simulink model "SKKPmdl"  (Simulink 8.4)
settings: Solver=ode113  StartTime=0.0  StopTime=900  FixedStep=0.1  RelTol=1e-1  AbsTol=1e-1
undefined symbols (not defined in the file or in its folder): deg, eps_max, eps_min, H3dm, H4dm, Jdm, L, M3dm, M4dm, Newton, P, R0, rad, Raphson, s, Td, Tpp, V0, y_out
libraries: aerolibconvert2 x26, aerolibtransform2 x19, aerolibutil x7, aerolibobsolete x6, dspinverses x5, vrlib x1, aerolib6dof2 x1
(part 1 of 2)
settings Model: Creator=Mikhail  LastModifiedBy=Mikhail  PauseTimes=1  BufferReuse=off
settings DataIOCC: SignalLoggingSaveFormat=Dataset
settings OptimizationCC: BlockReduction=off  InlineParams=on  BufferReuse=off  ExpressionDepthLimit=128
settings DebuggingCC: UnderspecifiedInitializationDetection=Simplified  MergeDetectMultiDrivingBlocksExec=error  FcnCallInpInsideContextMsg=EnableAllAsError  StateNameClashWarn=none
settings GRTTargetCC: CombineOutputUpdateFcns=on  GRTInterface=off

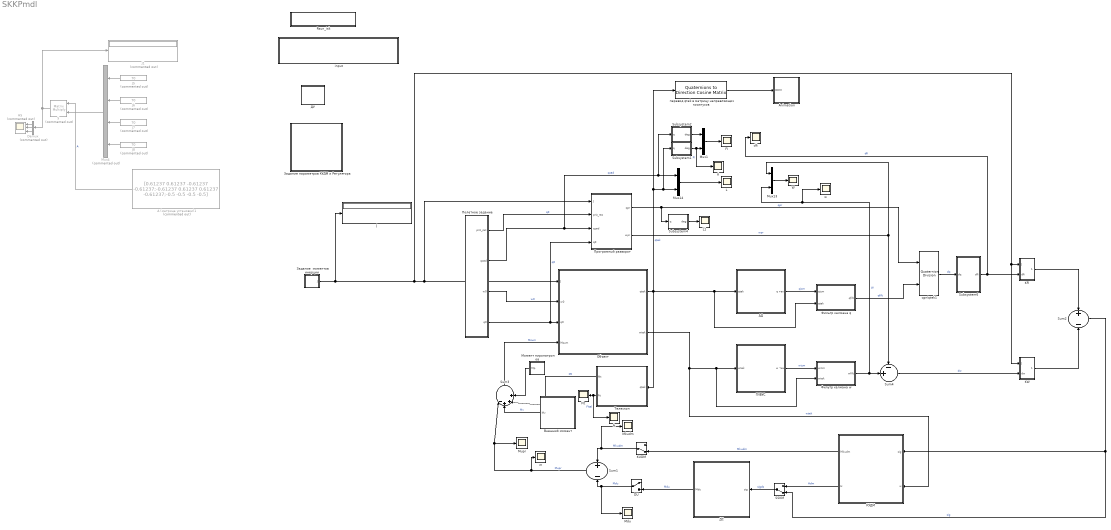
== system SKKPmdl ==
  " 5" : Product  Commented=on  Multiplication=Matrix(*)
  Animation : Subsystem  AncestorBlock=aerolibanim/6DoF Animation  mask(Animation){u2=10, u8=off}
      mask prompts: u2 "Time interval between updates:"; u8 "Enable animation"
      mask help: Create a 3-D animated.
      mask init:
      | Config.update = u2;
      | Config.Animenable = u8;
      mask Help: web(asbhelp('6dofanimation'));
  DU : ManualSwitch
  Demux : Demux  Commented=on  Outputs=3
  FI : Scope
      settings: TickLabels=on  YMax=30  SaveName=FI  SampleInput=on  ScrollMode=on
  FIt : Scope
      settings: YMin=-20  YMax=100  SaveName=FIt
  H5 : Scope  Commented=on  NumInputPorts=3
      settings: TimeRange=250  YMin=-100~-5~-5  YMax=600~5~5  SaveName=H4dm3
  J : Display
  J1 : Display  Commented=on
  J{5..8} (4 alike) : Constant  Commented=on  Value=70
  KFI : Subsystem
  KUDM : ManualSwitch  CurrentSetting=0
  KW : Subsystem
  L : Scope
      settings: YMin=0  YMax=1  SaveName=L
  L1 : Scope
      settings: YMin=0  YMax=8  SaveName=L1
  Mdu : Scope
      settings: YMin=-0.2  YMax=1  SaveName=Mdu
  Mkudm : Scope
      settings: YMin=-0.25  YMax=0.05  SaveName=Mkudm
  Mupr : Scope
      settings: YMin=-0.1  YMax=0.6  SaveName=Mupr
  Mux1 : Mux  Inputs=2
  Mux13 : Mux  Inputs=2
  Mux14 : Mux  Inputs=2
  Mux4 : Mux  Commented=on
  "Rsun_isk " : Subsystem  mask{rsun=[3 50 0]'}
      mask init:
      | Rsun=rsun/(norm(rsun));
      | assignin('base','Rsun',Rsun);
      | st=sprintf('Rsun=[%1.2g %1.2g %1.2g]\n',Rsun);
      mask Display: disp(st);
  SSKM : ManualSwitch  CurrentSetting=0
  Subsystem1 : Subsystem
  Subsystem2 : Subsystem
  Subsystem4 : Subsystem
  Subsystem6 : Subsystem
  Sum1 : Sum  Inputs=+-
  Sum2 : Sum  Inputs=+-
  Sum3 : Sum  Inputs=|-+++
  Sum4 : Sum  Inputs=-+|
  W : Scope
      settings: TimeRange=350  YMin=-50  YMax=250  SaveName=W
  dfi : Scope
      settings: YMin=-0.2  YMax=0.1  SaveName=dfi
  fi : Scope
      settings: ShowLegends=on  YMax=35  SaveName=ScopeData2
  ft : Scope
      settings: ShowLegends=on  YMin=-50  YMax=200  SaveName=ScopeData8
  input : Subsystem  mask{P=1, L=1.5, Td=0.1, X=0.006, Y=1.229, Z=-0.001}
      mask init:
      | assignin('base','P',P);
      | assignin('base','L',L);
      | assignin('base','Td',Td);
      | assignin('base','X',X);
      | assignin('base','Y',Y);
      | assignin('base','Z',Z);
      | 
      | st=sprintf('Тяга P =%1.3fН\n Плечо L =%1.3fм\n Постоянная времени нарастания/спада  Td =%1.3fc\n',P,L,Td);
      mask Callback P:
      | %assignin('base','psi0',psi0);
      | %assignin('base','tetta0',tetta0);
      mask Display: disp(st);
  m : Scope
      settings: ShowLegends=on  TimeRange=14.16568047337279  YMin=0.2  YMax=0.45  SaveName=ScopeData7
  qpr/qtek1 : aerolibutil/Quaternion Division
  w : Scope
      settings: ShowLegends=on  YMin=0  YMax=0.2  SaveName=ScopeData5
  А (матрица установки)1 : Constant  Commented=on  Value=[0.61237 0.61237 -0.61237 -0.61237;-0.61237 0.61237 0.61237 -0.61237;-0.5 -0.5 -0.5 -0.5]
  АД : Subsystem
      mask Display: image(imread('AD.png'))
  Внешний момент : Subsystem
  ГИВУС : Subsystem
      mask Display: image(imread('GIVUS.jpg'))
  ДC : Subsystem
      mask Display: image(imread('DS.jpg'))
  ДУ : Subsystem  mask{eps_min=1, eps_max=0.1, y_out=1}
      mask prompts: eps_min "Порог включения"; eps_max "Порог отключения"; y_out "Выходной сигнал"
      mask init:
      | assignin('base','eps_min',eps_min);
      | assignin('base','eps_max',eps_max);
      | assignin('base','y_out',y_out);
      mask Display:
      | plot([0.1 0.9],[0.5 0.5]);
      | plot([0.5 0.5],[0.1 0.9]);
      | plot([0.1 0.4 0.4 0.6 0.6 0.9],[0.3 0.3 0.5 0.5 0.7 0.7])
      | plot([0.1 0.45 0.45 0.55 0.55 0.9],[0.3 0.3 0.5 0.5 0.7 0.7])
  Задание  моментов инерции : Subsystem
  Задание параметров КУДМ и Регулятора : Subsystem  mask{jdm=0.0634646, tpp=50, e=0.8, m3dm=0.3, m4dm=0.4, h3dm=43, h4dm=140}
      mask init:
      | Jdm=jdm;
      | Tpp=tpp;
      | E=e;
      | M3dm=m3dm;
      | M4dm=m4dm;
      | H3dm=h3dm;
      | H4dm=h4dm;
      | 
      | assignin('base','Jdm',Jdm);
      | 
      | assignin('base','Tpp',Tpp);
      | assignin('base','E',E);
      | 
      | assignin('base','M3dm',M3dm);
      | assignin('base','M4dm',M4dm);
      | 
      | assignin('base','H3dm',H3dm);
      | assignin('base','H4dm',H4dm);
      | 
      | st=sprintf('Jdm=%g\n Tpp=%g\n E=%g\n M3dm=%g\n M4dm=%g\n H3dm=%g\n H4dm=%g\n',jdm,tpp,e,m3dm,m4dm,h3dm,h4dm);
      mask Display: disp(st);
  КУДМ : Subsystem
      mask Display: image(imread('KUDM.jpg'))
  Момент пиропатронов : Subsystem
  Объект : Subsystem
      mask Display: image(imread('КА.png'))
  Полетное задание : Subsystem
  "Програмный разворот " : Subsystem
  Телескоп : Subsystem
      mask Display: image(imread('Tel.png'))
  "Фильтр калмана q " : Subsystem
  "Фильтр калмана w " : Subsystem
  "перевод qtek в матрицу направляющих косинусов " : aerolibtransform2/Quaternions to  Direction Cosine Matrix
  wires:
  "Програмный разворот "/1(qpr) -> Subsystem4/1(q), qpr/qtek1/1  "qpr"
  Объект/2(wtek) -> КУДМ/2(w), "Фильтр калмана w "/2(wtek), ГИВУС/1(wtek)  "wtek"
  ГИВУС/1(w тек) -> "Фильтр калмана w "/1(wizm)  "wizm"
  Объект/1(qtek) -> "Фильтр калмана q "/2(qtek), АД/1("qtek "), Телескоп/1(qtek), "перевод qtek в матрицу направляющих косинусов "/1, Subsystem1/1(q), Mux14/2  "qtek"
  АД/1(q тек) -> "Фильтр калмана q "/1(qizm)  "qizm"
  Полетное задание/3(w0) -> Объект/2(w0)  "w0"
  qpr/qtek1/1 -> Subsystem6/1(dq)  "dq"
  Subsystem6/1(dfi) -> dfi/1, KFI/2(dfi)  "dfi"
  Sum2/1 -> SSKM/2, КУДМ/1(sig)  "sig"
  КУДМ/2(H) -> SSKM/1  "Hdm"
  SSKM/1 -> ДC/1(sig)  "sigds"
  ДC/1(Mdu) -> DU/2  "Mdu"
  КУДМ/1(Mkudm) -> KUDM/2  "Mkudm"
  Внешний момент/1("Mv ") -> Sum3/2  "Mv"
  Sum1/1 -> m/1, Mupr/1, Sum3/1  "Mupr"
  Sum3/1 -> Объект/4(Msum)  "Msum"
  "Фильтр калмана q "/1(qfilt) -> qpr/qtek1/2  "qfilt"
  Mux14/1 -> L/1
  "Програмный разворот "/2(wpr) -> Sum4/1, Mux13/1  "wpr"
  Mux13/1 -> W/1
  "Фильтр калмана w "/1(wfilt) -> w/1, Mux13/2, Sum4/2  "W"
  KUDM/1 -> Mkudm/1, Sum1/1  "Mkudm"
  DU/1 -> Mdu/1, Sum1/2  "Mdu"
  Subsystem1/1(deg) -> fi/1, Mux1/2  "FI"
  Subsystem2/1(deg) -> Mux1/1
  Mux1/1 -> FI/1
  "перевод qtek в матрицу направляющих косинусов "/1 -> Animation/1(DCM)
  Полетное задание/4(q0) -> "Програмный разворот "/4(q0), Объект/3("q0 ")  "q0"
  Subsystem4/1(deg) -> L1/1
  Полетное задание/1(priz_raz) -> "Програмный разворот "/2(priz_raz)  "q0"
  Полетное задание/2(qzad) -> Subsystem2/1(q), Mux14/1, "Програмный разворот "/3(qzad)  "qzad"
  Телескоп/1(Mt) -> Sum3/3  "Mt"
  Телескоп/2(fit) -> ft/1, FIt/1  "FItel"
  Задание  моментов инерции/1(J) -> "Програмный разворот "/1(J), Объект/1(J), KW/1(J), KFI/1(J), J/1
  Момент пиропатронов/1(Mp) -> Sum3/4
  KFI/1(kfi*dfi) -> Sum2/1
  Sum4/1 -> KW/2(dw)  "dw"
  KW/1(kw*dw) -> Sum2/2
  J5/1 -> Mux4/1
  J6/1 -> Mux4/2
  J7/1 -> Mux4/3
  J8/1 -> Mux4/4
  Mux4/1 -> " 5"/2
  " 5"/1 -> Demux/1, J1/1
  Demux/1 -> H5/1
  Demux/2 -> H5/2
  Demux/3 -> H5/3
  А (матрица установки)1/1 -> " 5"/1  "A"

== system SKKPmdl/Animation ==
  DCM : Inport
  Animation S-Function : S-Function  FunctionName=saeroanim  Parameters=Config  EnableBusSupport=off
  Reshape : Reshape
  wires:
  DCM/1 -> Reshape/1
  Reshape/1 -> Animation S-Function/1

== system SKKPmdl/KFI ==
  J : Inport
  dfi : Inport  Port=2
  Demux : Demux  Outputs=9
  Display4 : Display
  Divide1 : Product  Inputs=**
  Divide3 : Product  Inputs=/*
  Divide4 : Product  Inputs=/*
  Divide5 : Product  Inputs=/*
  Mux : Mux  Inputs=3
  Reshape : Reshape  OutputDimensionality=Column vector (2-D)
  eps_max3 : Constant  Value=Tpp*Tpp
  kfi*dfi : Outport
  wires:
  Divide1/1 -> kfi*dfi/1  "kfi*dfi"
  Demux/5 -> Divide4/2
  eps_max3/1 -> Divide5/1, Divide4/1, Divide3/1
  Demux/9 -> Divide5/2
  Divide3/1 -> Mux/1
  Divide4/1 -> Mux/2
  Divide5/1 -> Mux/3
  Demux/1 -> Divide3/2
  Reshape/1 -> Demux/1
  Mux/1 -> Divide1/1, Display4/1
  dfi/1 -> Divide1/2
  J/1 -> Reshape/1

== system SKKPmdl/KW ==
  J : Inport
  dw : Inport  Port=2
  Demux1 : Demux  Outputs=9
  Display5 : Display
  Divide{2,6..8} (4 alike) : Product  Inputs=**
  Mux2 : Mux  Inputs=3
  Reshape1 : Reshape  OutputDimensionality=Column vector (2-D)
  eps_max1 : Constant  Value=(2*E)/Tpp
  kw*dw : Outport
  wires:
  dw/1 -> Divide2/2
  Divide2/1 -> kw*dw/1  "kw*dw"
  Demux1/1 -> Divide6/2
  Demux1/9 -> Divide8/2
  eps_max1/1 -> Divide6/1, Divide7/1, Divide8/1
  Demux1/5 -> Divide7/2
  Divide6/1 -> Mux2/1
  Divide7/1 -> Mux2/2
  Divide8/1 -> Mux2/3
  Reshape1/1 -> Demux1/1
  Mux2/1 -> Display5/1, Divide2/1
  J/1 -> Reshape1/1

== system SKKPmdl/Rsun_isk  ==

== system SKKPmdl/Subsystem1 ==
  q : Inport
  Angle Conversion1 : aerolibconvert2/Angle Conversion  IU=rad  OU=deg
  Direction Cosine Matrix to Euler Angles1 : aerolibobsolete/Direction Cosine Matrix to Euler Angles
  Quaternions to  Direction Cosine Matrix3 : aerolibtransform2/Quaternions to  Direction Cosine Matrix
  deg : Outport
  wires:
  Quaternions to  Direction Cosine Matrix3/1 -> Direction Cosine Matrix to Euler Angles1/1
  Direction Cosine Matrix to Euler Angles1/1 -> Angle Conversion1/1
  Angle Conversion1/1 -> deg/1
  q/1 -> Quaternions to  Direction Cosine Matrix3/1

== system SKKPmdl/Subsystem2 ==
  q : Inport
  Angle Conversion1 : aerolibconvert2/Angle Conversion  IU=rad  OU=deg
  Direction Cosine Matrix to Euler Angles1 : aerolibobsolete/Direction Cosine Matrix to Euler Angles
  Quaternions to  Direction Cosine Matrix3 : aerolibtransform2/Quaternions to  Direction Cosine Matrix
  deg : Outport
  wires:
  q/1 -> Quaternions to  Direction Cosine Matrix3/1
  Angle Conversion1/1 -> deg/1
  Direction Cosine Matrix to Euler Angles1/1 -> Angle Conversion1/1
  Quaternions to  Direction Cosine Matrix3/1 -> Direction Cosine Matrix to Euler Angles1/1

== system SKKPmdl/Subsystem4 ==
  q : Inport
  Angle Conversion1 : aerolibconvert2/Angle Conversion  IU=rad  OU=deg
  Direction Cosine Matrix to Euler Angles1 : aerolibobsolete/Direction Cosine Matrix to Euler Angles
  Quaternions to  Direction Cosine Matrix3 : aerolibtransform2/Quaternions to  Direction Cosine Matrix
  deg : Outport
  wires:
  Quaternions to  Direction Cosine Matrix3/1 -> Direction Cosine Matrix to Euler Angles1/1
  Direction Cosine Matrix to Euler Angles1/1 -> Angle Conversion1/1
  Angle Conversion1/1 -> deg/1
  q/1 -> Quaternions to  Direction Cosine Matrix3/1

== system SKKPmdl/Subsystem6 ==
  dq : Inport
  Angle C5 : aerolibconvert2/Angle Conversion  IU=rad  OU=deg
  Перевод из матрицы направляющих косинусов  в dfi1 : aerolibobsolete/Direction Cosine Matrix to Euler Angles
  перевод dq в матрицу направляющих косинусов 1 : aerolibtransform2/Quaternions to  Direction Cosine Matrix
  dfi : Outport
  wires:
  перевод dq в матрицу направляющих косинусов 1/1 -> Перевод из матрицы направляющих косинусов  в dfi1/1  "DCM"
  dq/1 -> перевод dq в матрицу направляющих косинусов 1/1
  Перевод из матрицы направляющих косинусов  в dfi1/1 -> Angle C5/1  "dfi"
  Angle C5/1 -> dfi/1

== system SKKPmdl/input ==

== system SKKPmdl/АД ==
  "qtek " : Inport
  Gain3 : Gain  Gain=3
  Gain4 : Gain  Gain=3
  Gain5 : Gain  Gain=3
  Mux2 : Mux  Inputs=3
  Noise1____5''1 : RandomNumber  Variance=0.0013888888888889  Seed=23456
  Noise2___5''1 : RandomNumber  Variance=0.0013888888888889  Seed=23455
  Noise3___5''1 : RandomNumber  Variance=0.0013888888888889  Seed=23457
  Quaternion Multiplication3 : aerolibutil/Quaternion Multiplication
  Quaternion Multiplication4 : aerolibutil/Quaternion Multiplication
  Quaternion Multiplication5 : aerolibutil/Quaternion Multiplication
  Zero-Order Hold8 : ZeroOrderHold  SampleTime=0.1
  Мвск-пск 1 : Constant  Value=[0 0 1;-0.5 0.87 0;-0.87 -0.5 0]
  Мпск-вск1 : Constant  Value=[0 -0.5 -0.85; 0 0.85 -0.5; 1 0 0]
  Перевод из матрицы  направляющих  косинусов в  кватернионы2 : aerolibtransform2/Direction Cosine Matrix  to Quaternions
  Перевод из матрицы  направляющих  косинусов в  кватернионы3 : aerolibtransform2/Direction Cosine Matrix  to Quaternions
  Перевод из углов  в кватернионы1 : Subsystem
  q тек : Outport
  wires:
  Мвск-пск 1/1 -> Перевод из матрицы  направляющих  косинусов в  кватернионы2/1  "Mвск-пск"
  Noise1____5''1/1 -> Gain3/1
  Noise2___5''1/1 -> Gain4/1
  Noise3___5''1/1 -> Gain5/1
  Mux2/1 -> Перевод из углов  в кватернионы1/1(fi)
  "qtek "/1 -> Quaternion Multiplication3/2  "qtek"
  Перевод из матрицы  направляющих  косинусов в  кватернионы2/1 -> Quaternion Multiplication3/1
  Перевод из углов  в кватернионы1/1(q) -> Quaternion Multiplication4/2  "Добавление шумовой составляющей АД"
  Мпск-вск1/1 -> Перевод из матрицы  направляющих  косинусов в  кватернионы3/1  "Mпск-вск"
  Quaternion Multiplication4/1 -> Quaternion Multiplication5/2
  Quaternion Multiplication5/1 -> q тек/1
  Перевод из матрицы  направляющих  косинусов в  кватернионы3/1 -> Quaternion Multiplication5/1
  Gain3/1 -> Mux2/1
  Gain4/1 -> Mux2/2
  Gain5/1 -> Mux2/3
  Quaternion Multiplication3/1 -> Quaternion Multiplication4/1

== system SKKPmdl/Внешний момент ==
  M_vn4 : Step  Time=0  After=0.00001  SampleTime=0
  M_vn5 : Step  Time=0  After=0.00008  SampleTime=0
  M_vn6 : Step  Time=0  After=0.00006  SampleTime=0
  Mux4 : Mux  Inputs=3
  "Mv " : Outport
  wires:
  M_vn4/1 -> Mux4/1
  M_vn6/1 -> Mux4/3
  M_vn5/1 -> Mux4/2
  Mux4/1 -> "Mv "/1

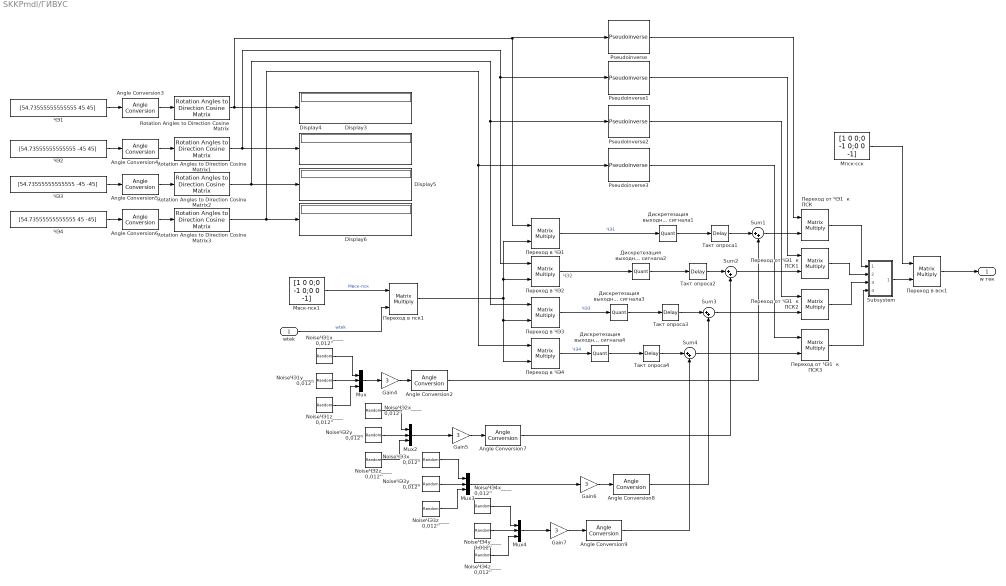
== system SKKPmdl/ГИВУС ==
  note: ЧЭ2
  wtek : Inport
  Angle Conversion{2..9} (8 alike) : aerolibconvert2/Angle Conversion  IU=deg  OU=rad
  Display{3..6} (4 alike) : Display
  Gain{4..7} (4 alike) : Gain  Gain=3
  Mux{,2..4} (4 alike) : Mux  Inputs=3
  NoiseЧЭ1x____0,012'' : RandomNumber  Variance=0.0000033333333333333  Seed=23456
  NoiseЧЭ1y____0,012'' : RandomNumber  Variance=0.0000033333333333333  Seed=23456
  NoiseЧЭ1z____0,012'' : RandomNumber  Variance=0.0000033333333333333  Seed=23456
  NoiseЧЭ2x____0,012'' : RandomNumber  Variance=0.0000033333333333333  Seed=23456
  NoiseЧЭ2y____0,012'' : RandomNumber  Variance=0.0000033333333333333  Seed=23456
  NoiseЧЭ2z____0,012'' : RandomNumber  Variance=0.0000033333333333333  Seed=23456
  NoiseЧЭ3x____0,012'' : RandomNumber  Variance=0.0000033333333333333  Seed=23456
  NoiseЧЭ3y____0,012'' : RandomNumber  Variance=0.0000033333333333333  Seed=23456
  NoiseЧЭ3z____0,012'' : RandomNumber  Variance=0.0000033333333333333  Seed=23456
  NoiseЧЭ4x____0,012'' : RandomNumber  Variance=0.0000033333333333333  Seed=23456
  NoiseЧЭ4y____0,012'' : RandomNumber  Variance=0.0000033333333333333  Seed=23456
  NoiseЧЭ4z____0,012'' : RandomNumber  Variance=0.0000033333333333333  Seed=23456
  Pseudoinverse{,1..3} (4 alike) : dspinverses/Pseudoinverse  wanterr=off
  Rotation Angles to Direction Cosine Matrix{,1..3} (4 alike) : aerolibtransform2/Rotation Angles to Direction Cosine Matrix  rotationOrder=XYZ
  Subsystem : Subsystem
  Sum{1..4} (4 alike) : Sum  Inputs=|++
  Дискретезация выходного сигнала{1..4} (4 alike) : Quantizer  QuantizationInterval=0.000000048481368110954
  Мвск-пск1 : Constant  Value=[1 0 0;0 -1 0;0 0 -1]  VectorParams1D=off
  Мпск-сск : Constant  Value=[1 0 0;0 -1 0;0 0 -1]  VectorParams1D=off
  Переход в ЧЭ{1..4} (4 alike) : Product  Multiplication=Matrix(*)  SaturateOnIntegerOverflow=on  RndMeth=Zero  InputSameDT=on  OutDataTypeStr=Inherit: Same as first input
  Переход в вск1 : Product  Multiplication=Matrix(*)  SaturateOnIntegerOverflow=on  RndMeth=Zero  InputSameDT=on  OutDataTypeStr=Inherit: Same as first input
  Переход в пск1 : Product  Multiplication=Matrix(*)  SaturateOnIntegerOverflow=on  RndMeth=Zero  InputSameDT=on  OutDataTypeStr=Inherit: Same as first input
  Переход от ЧЭ1  к ПСК{,1..3} (4 alike) : Product  Multiplication=Matrix(*)  SaturateOnIntegerOverflow=on  RndMeth=Zero  InputSameDT=on  OutDataTypeStr=Inherit: Same as first input
  Такт опроса{1..4} (4 alike) : TransportDelay  DelayTime=0.1
  ЧЭ1 : Constant  Value=[54.73555555555555 45 45]
  ЧЭ2 : Constant  Value=[54.73555555555555 -45 45]
  ЧЭ3 : Constant  Value=[54.73555555555555 -45 -45]
  ЧЭ4 : Constant  Value=[54.73555555555555 45 -45]
  w тек : Outport
  wires:
  Мпск-сск/1 -> Переход в вск1/1
  Мвск-пск1/1 -> Переход в пск1/1  "Mвск-пск"
  wtek/1 -> Переход в пск1/2  "wtek"
  NoiseЧЭ1x____0,012''/1 -> Mux/1
  Gain4/1 -> Angle Conversion2/1
  Переход в вск1/1 -> w тек/1
  Gain5/1 -> Angle Conversion7/1
  Gain6/1 -> Angle Conversion8/1
  Gain7/1 -> Angle Conversion9/1
  Angle Conversion3/1 -> Rotation Angles to Direction Cosine Matrix/1
  ЧЭ1/1 -> Angle Conversion3/1
  Rotation Angles to Direction Cosine Matrix/1 -> Display3/1, Переход в ЧЭ1/1, Pseudoinverse/1
  Angle Conversion4/1 -> Rotation Angles to Direction Cosine Matrix1/1
  ЧЭ2/1 -> Angle Conversion4/1
  Rotation Angles to Direction Cosine Matrix1/1 -> Display4/1, Pseudoinverse1/1, Переход в ЧЭ2/1
  Angle Conversion5/1 -> Rotation Angles to Direction Cosine Matrix2/1
  ЧЭ3/1 -> Angle Conversion5/1
  Rotation Angles to Direction Cosine Matrix2/1 -> Display5/1, Pseudoinverse2/1, Переход в ЧЭ3/1
  Angle Conversion6/1 -> Rotation Angles to Direction Cosine Matrix3/1
  ЧЭ4/1 -> Angle Conversion6/1
  Rotation Angles to Direction Cosine Matrix3/1 -> Display6/1, Pseudoinverse3/1, Переход в ЧЭ4/1
  Переход в пск1/1 -> Переход в ЧЭ4/2, Переход в ЧЭ3/2, Переход в ЧЭ2/2, Переход в ЧЭ1/2
  Такт опроса1/1 -> Sum1/1
  Дискретезация выходного сигнала1/1 -> Такт опроса1/1
  Такт опроса2/1 -> Sum2/1
  Дискретезация выходного сигнала2/1 -> Такт опроса2/1
  Такт опроса3/1 -> Sum3/1
  Дискретезация выходного сигнала3/1 -> Такт опроса3/1
  Такт опроса4/1 -> Sum4/1
  Дискретезация выходного сигнала4/1 -> Такт опроса4/1
  Переход в ЧЭ4/1 -> Дискретезация выходного сигнала4/1  "ЧЭ4"
  Переход в ЧЭ3/1 -> Дискретезация выходного сигнала3/1  "ЧЭ3"
  Переход в ЧЭ2/1 -> Дискретезация выходного сигнала2/1
  Переход в ЧЭ1/1 -> Дискретезация выходного сигнала1/1  "ЧЭ1"
  Angle Conversion2/1 -> Sum1/2
  Angle Conversion7/1 -> Sum2/2
  Angle Conversion8/1 -> Sum3/2
  Angle Conversion9/1 -> Sum4/2
  Sum1/1 -> Переход от ЧЭ1  к ПСК/2
  Sum4/1 -> Переход от ЧЭ1  к ПСК3/2
  Sum3/1 -> Переход от ЧЭ1  к ПСК2/2
  Sum2/1 -> Переход от ЧЭ1  к ПСК1/2
  Pseudoinverse/1 -> Переход от ЧЭ1  к ПСК/1
  Pseudoinverse1/1 -> Переход от ЧЭ1  к ПСК1/1
  Pseudoinverse2/1 -> Переход от ЧЭ1  к ПСК2/1
  Pseudoinverse3/1 -> Переход от ЧЭ1  к ПСК3/1
  Mux/1 -> Gain4/1
  NoiseЧЭ1z____0,012''/1 -> Mux/3
  NoiseЧЭ1y____0,012''/1 -> Mux/2
  NoiseЧЭ2x____0,012''/1 -> Mux2/1
  Mux2/1 -> Gain5/1
  NoiseЧЭ2z____0,012''/1 -> Mux2/3
  NoiseЧЭ2y____0,012''/1 -> Mux2/2
  NoiseЧЭ3x____0,012''/1 -> Mux3/1
  Mux3/1 -> Gain6/1
  NoiseЧЭ3z____0,012''/1 -> Mux3/3
  NoiseЧЭ3y____0,012''/1 -> Mux3/2
  NoiseЧЭ4x____0,012''/1 -> Mux4/1
  Mux4/1 -> Gain7/1
  NoiseЧЭ4z____0,012''/1 -> Mux4/3
  NoiseЧЭ4y____0,012''/1 -> Mux4/2
  Переход от ЧЭ1  к ПСК1/1 -> Subsystem/2(ЧЭ2)
  Переход от ЧЭ1  к ПСК2/1 -> Subsystem/3(ЧЭ3)
  Переход от ЧЭ1  к ПСК3/1 -> Subsystem/4(ЧЭ4)
  Переход от ЧЭ1  к ПСК/1 -> Subsystem/1(ЧЭ1)
  Subsystem/1(wпск) -> Переход в вск1/2

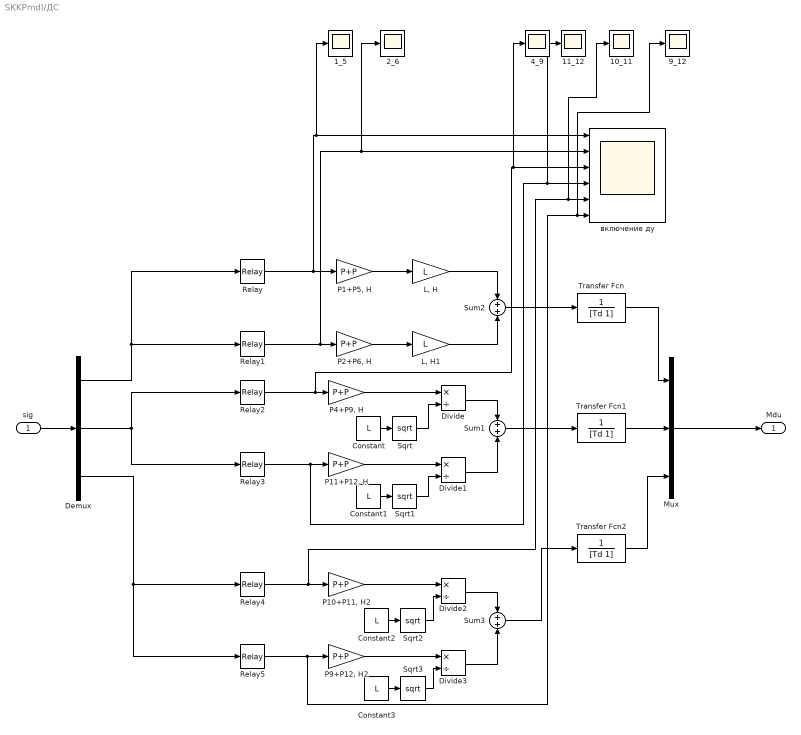
== system SKKPmdl/ДC ==
  sig : Inport
  10_11 : Scope
      settings: SaveName=P1011
  11_12 : Scope
      settings: SaveName=P1112
  1_5 : Scope
      settings: YMin=0  YMax=1  SaveName=P15
  2_6 : Scope
      settings: YMin=-1  YMax=0  SaveName=P26
  4_9 : Scope
      settings: SaveName=P49
  9_12 : Scope
      settings: SaveName=P912
  Constant{,1..3} (4 alike) : Constant  Value=L
  Demux : Demux  Outputs=3
  Divide{,1..3} (4 alike) : Product  Inputs=*/
  "L, Н" : Gain  Gain=L  SaturateOnIntegerOverflow=on  OutDataTypeStr=Inherit: Same as input  ParamDataTypeStr=Inherit: Same as input
  "L, Н1" : Gain  Gain=L  SaturateOnIntegerOverflow=on  OutDataTypeStr=Inherit: Same as input  ParamDataTypeStr=Inherit: Same as input
  Mux : Mux  Inputs=3
  "P1+P5, Н" : Gain  Gain=P+P  SaturateOnIntegerOverflow=on  OutDataTypeStr=Inherit: Same as input  ParamDataTypeStr=Inherit: Same as input
  "P10+P11, Н2" : Gain  Gain=P+P  SaturateOnIntegerOverflow=on  OutDataTypeStr=Inherit: Same as input  ParamDataTypeStr=Inherit: Same as input
  "P11+P12, Н" : Gain  Gain=P+P  SaturateOnIntegerOverflow=on  OutDataTypeStr=Inherit: Same as input  ParamDataTypeStr=Inherit: Same as input
  "P2+P6, Н" : Gain  Gain=P+P  SaturateOnIntegerOverflow=on  OutDataTypeStr=Inherit: Same as input  ParamDataTypeStr=Inherit: Same as input
  "P4+P9, Н" : Gain  Gain=P+P  SaturateOnIntegerOverflow=on  OutDataTypeStr=Inherit: Same as input  ParamDataTypeStr=Inherit: Same as input
  "P9+P12, Н2" : Gain  Gain=P+P  SaturateOnIntegerOverflow=on  OutDataTypeStr=Inherit: Same as input  ParamDataTypeStr=Inherit: Same as input
  Relay : Relay  OnSwitchValue=eps_min  OffSwitchValue=eps_max  OnOutputValue=y_out
  Relay1 : Relay  OnSwitchValue=-eps_max  OffSwitchValue=-eps_min  OnOutputValue=0  OffOutputValue=-y_out
  Relay2 : Relay  OnSwitchValue=eps_min  OffSwitchValue=eps_max  OnOutputValue=y_out
  Relay3 : Relay  OnSwitchValue=-eps_max  OffSwitchValue=-eps_min  OnOutputValue=0  OffOutputValue=-y_out
  Relay4 : Relay  OnSwitchValue=eps_min  OffSwitchValue=eps_max  OnOutputValue=y_out
  Relay5 : Relay  OnSwitchValue=-eps_max  OffSwitchValue=-eps_min  OnOutputValue=0  OffOutputValue=-y_out
  Sqrt{,1..3} (4 alike) : Sqrt  SaturateOnIntegerOverflow=on
  Sum1 : Sum
  Sum2 : Sum
  Sum3 : Sum
  Transfer Fcn : TransferFcn  Denominator=[Td 1]
  Transfer Fcn1 : TransferFcn  Denominator=[Td 1]
  Transfer Fcn2 : TransferFcn  Denominator=[Td 1]
  включение ду : Scope  NumInputPorts=6
      settings: TimeRange=500  YMin=-1~-1~-1~-1~-1~-1  YMax=1~1~1~1~1~1  SaveName=M12
  Mdu : Outport
  wires:
  Sqrt2/1 -> Divide2/2
  Constant2/1 -> Sqrt2/1
  Constant3/1 -> Sqrt3/1
  Sqrt3/1 -> Divide3/2
  Constant1/1 -> Sqrt1/1
  Sqrt1/1 -> Divide1/2
  Sqrt/1 -> Divide/2
  Constant/1 -> Sqrt/1
  Relay5/1 -> "P9+P12, Н2"/1, включение ду/6, 9_12/1
  Transfer Fcn/1 -> Mux/1
  Sum2/1 -> Transfer Fcn/1
  Demux/1 -> Relay/1, Relay1/1
  Relay/1 -> "P1+P5, Н"/1, включение ду/1, 1_5/1
  sig/1 -> Demux/1
  Sum1/1 -> Transfer Fcn1/1
  Demux/2 -> Relay2/1, Relay3/1
  Relay2/1 -> "P4+P9, Н"/1, включение ду/3, 4_9/1
  Transfer Fcn1/1 -> Mux/2
  Sum3/1 -> Transfer Fcn2/1
  Relay4/1 -> "P10+P11, Н2"/1, включение ду/5, 10_11/1
  Transfer Fcn2/1 -> Mux/3
  Demux/3 -> Relay5/1, Relay4/1
  Relay1/1 -> "P2+P6, Н"/1, включение ду/2, 2_6/1
  Relay3/1 -> "P11+P12, Н"/1, включение ду/4, 11_12/1
  "P1+P5, Н"/1 -> "L, Н"/1
  "L, Н"/1 -> Sum2/1
  "P2+P6, Н"/1 -> "L, Н1"/1
  "L, Н1"/1 -> Sum2/2
  "P11+P12, Н"/1 -> Divide1/1
  Divide1/1 -> Sum1/2
  "P4+P9, Н"/1 -> Divide/1
  Divide/1 -> Sum1/1
  Divide3/1 -> Sum3/2
  Divide2/1 -> Sum3/1
  "P9+P12, Н2"/1 -> Divide3/1
  "P10+P11, Н2"/1 -> Divide2/1
  Mux/1 -> Mdu/1

== system SKKPmdl/ДУ ==

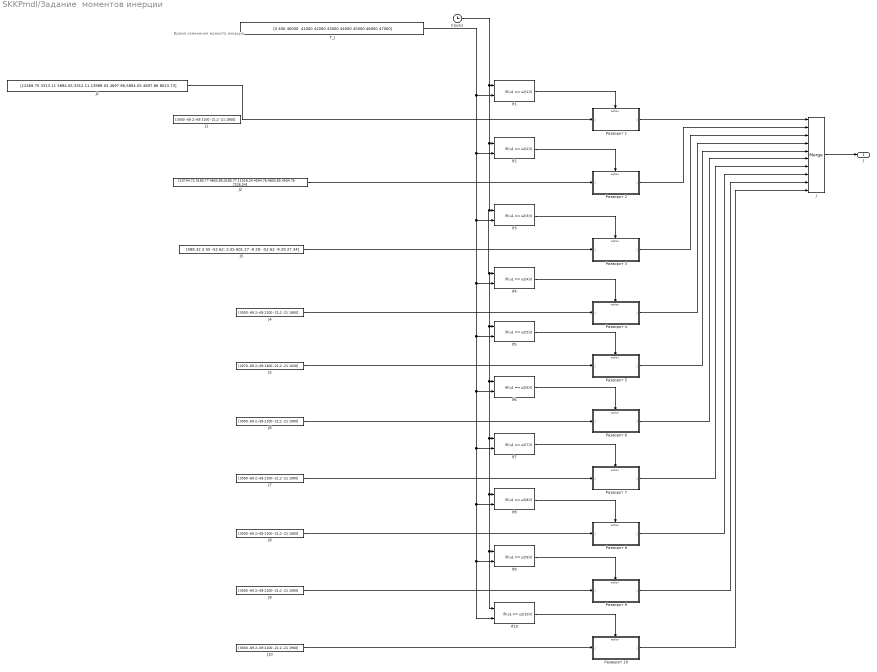
== system SKKPmdl/Задание  моментов инерции ==
  note: Время изменения момента инерции
  Clock1 : Clock
  If1 : If  NumInputs=2  IfExpression=(u1 == u2(1))  ShowElse=off
  If10 : If  NumInputs=2  IfExpression=(u1 == u2(10))  ShowElse=off
  If2 : If  NumInputs=2  IfExpression=(u1 == u2(2))  ShowElse=off
  If3 : If  NumInputs=2  IfExpression=(u1 == u2(3))  ShowElse=off
  If4 : If  NumInputs=2  IfExpression=(u1 == u2(4))  ShowElse=off
  If5 : If  NumInputs=2  IfExpression=(u1 == u2(5))  ShowElse=off
  If6 : If  NumInputs=2  IfExpression=(u1 == u2(6))  ShowElse=off
  If7 : If  NumInputs=2  IfExpression=(u1 == u2(7))  ShowElse=off
  If8 : If  NumInputs=2  IfExpression=(u1 == u2(8))  ShowElse=off
  If9 : If  NumInputs=2  IfExpression=(u1 == u2(9))  ShowElse=off
  J{1,4,6..10} (7 alike) : Constant  Value=[3500 -69 2;-69 2100 -21;2 -21 1900]
  "J1 " : Constant  Value=[12469.75 3313.11 5894.05;3312.11 13989.03 4697.86;5894.05 4697.86 8023.73]
  J2 : Constant  Value=[10734.72 3180.77 4803.85;3180.77 11518.24 4504.76;4803.85 4504.76 7226.24]
  J3 : Constant  Value=[588.32 2.55 -52.62; 2.55 601.27 -9.29; -52.62 -9.29 27.34]
  J5 : Constant  Value=[2070 -69 2;-69 1400 -21;2 -21 1030]
  T_j : Constant  Value="[0 400 40000  41000 42000 43000 44000 45000 46000 47000]"
  j : Merge  Inputs=10
  Разворот 1 : Subsystem  TreatAsAtomicUnit=on
  Разворот 10 : Subsystem  TreatAsAtomicUnit=on
  Разворот 2 : Subsystem  TreatAsAtomicUnit=on
  Разворот 3 : Subsystem  TreatAsAtomicUnit=on
  Разворот 4 : Subsystem  TreatAsAtomicUnit=on
  Разворот 5 : Subsystem  TreatAsAtomicUnit=on
  Разворот 6 : Subsystem  TreatAsAtomicUnit=on
  Разворот 7 : Subsystem  TreatAsAtomicUnit=on
  Разворот 8 : Subsystem  TreatAsAtomicUnit=on
  Разворот 9 : Subsystem  TreatAsAtomicUnit=on
  J : Outport
  wires:
  "J1 "/1 -> Разворот 1/1(j)
  If1/1 -> Разворот 1/Action
  J2/1 -> Разворот 2/1(j)
  If2/1 -> Разворот 2/Action
  J3/1 -> Разворот 3/1(j)
  If3/1 -> Разворот 3/Action
  J4/1 -> Разворот 4/1("j ")
  If4/1 -> Разворот 4/Action
  J5/1 -> Разворот 5/1("j ")
  If5/1 -> Разворот 5/Action
  J6/1 -> Разворот 6/1("j ")
  If6/1 -> Разворот 6/Action
  J7/1 -> Разворот 7/1("j ")
  If7/1 -> Разворот 7/Action
  J8/1 -> Разворот 8/1("j ")
  If8/1 -> Разворот 8/Action
  J9/1 -> Разворот 9/1("j ")
  If9/1 -> Разворот 9/Action
  J10/1 -> Разворот 10/1("j ")
  If10/1 -> Разворот 10/Action
  Разворот 1/1("j  ") -> j/1
  Разворот 2/1("j  ") -> j/2
  Разворот 3/1("j  ") -> j/3
  Разворот 4/1("j  ") -> j/4
  Разворот 5/1("j  ") -> j/5
  Разворот 6/1("j  ") -> j/6
  Разворот 7/1("j  ") -> j/7
  Разворот 8/1("j  ") -> j/8
  Разворот 9/1("j  ") -> j/9
  Разворот 10/1("j  ") -> j/10
  T_j/1 -> If2/2, If4/2, If6/2, If10/2, If9/2, If8/2, If7/2, If5/2, If3/2, If1/2
  Clock1/1 -> If10/1, If9/1, If8/1, If7/1, If6/1, If5/1, If4/1, If3/1, If2/1, If1/1
  j/1 -> J/1

== system SKKPmdl/Задание параметров КУДМ и Регулятора ==

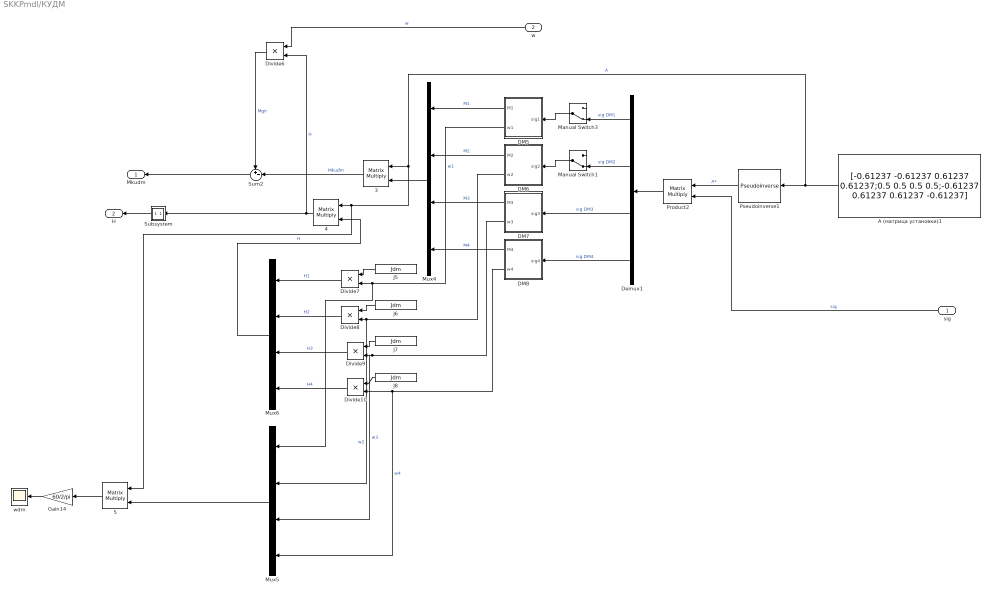
== system SKKPmdl/КУДМ ==
  sig : Inport
  w : Inport  Port=2
  " 3" : Product  Multiplication=Matrix(*)
  " 4" : Product  Multiplication=Matrix(*)
  " 5" : Product  Multiplication=Matrix(*)
  DM5 : Subsystem
  DM6 : Subsystem
  DM7 : Subsystem
  DM8 : Subsystem
  Demux1 : Demux
  Divide{6..10} (5 alike) : Product  Inputs=**
  Gain14 : Gain  Gain=60/2/pi
  J{5..8} (4 alike) : Constant  Value=Jdm
  Manual Switch1 : ManualSwitch  CurrentSetting=0
  Manual Switch3 : ManualSwitch  CurrentSetting=0
  Mux4 : Mux
  Mux5 : Mux
  Mux6 : Mux
  Product2 : Product  Multiplication=Matrix(*)  SaturateOnIntegerOverflow=on  OutDataTypeStr=Inherit: Same as first input
  Pseudoinverse1 : dspinverses/Pseudoinverse  wanterr=off
  Subsystem : Subsystem
  Sum2 : Sum  Inputs=+-|
  wdm : Scope
      settings: TimeRange=250  YMin=-2000  YMax=1500  SaveName=wdm
  А (матрица установки)1 : Constant  Value=[-0.61237 -0.61237 0.61237 0.61237;0.5 0.5 0.5 0.5;-0.61237 0.61237 0.61237 -0.61237]
  Mkudm : Outport
  H : Outport  Port=2
  wires:
  Gain14/1 -> wdm/1
  Subsystem/1(Out1) -> H/1
  Product2/1 -> Demux1/1
  DM7/1(M3) -> Mux4/3  "M3"
  w/1 -> Divide6/1  "w"
  Pseudoinverse1/1 -> Product2/1  "A*"
  А (матрица установки)1/1 -> Pseudoinverse1/1, " 5"/1, " 4"/1, " 3"/1  "A"
  DM8/1(M4) -> Mux4/4  "M4"
  Mux4/1 -> " 3"/2
  Mux6/1 -> " 4"/2  "H"
  " 3"/1 -> Sum2/2  "Mkudm"
  Divide6/1 -> Sum2/1  "Mgir"
  sig/1 -> Product2/2  "sig"
  DM5/2(w1) -> Mux5/1, Divide7/2  "w1"
  DM6/2(w2) -> Mux5/2, Divide8/2  "w2"
  Divide7/1 -> Mux6/1  "H1"
  Divide8/1 -> Mux6/2  "H2"
  Divide9/1 -> Mux6/3  "H3"
  Divide10/1 -> Mux6/4  "H4"
  DM7/2(w3) -> Mux5/3, Divide9/2  "w3"
  DM8/2(w4) -> Mux5/4, Divide10/2  "w4"
  J5/1 -> Divide7/1
  J6/1 -> Divide8/1
  J7/1 -> Divide9/1
  J8/1 -> Divide10/1
  DM5/1(M1) -> Mux4/1  "M1"
  Demux1/4 -> DM8/1(sig4)  "sig DM4"
  Demux1/3 -> DM7/1(sig3)  "sig DM3"
  DM6/1(M2) -> Mux4/2  "M2"
  Demux1/1 -> Manual Switch3/2  "sig DM1"
  " 4"/1 -> Divide6/2, Subsystem/1(In1)  "H"
  Demux1/2 -> Manual Switch1/2  "sig DM2"
  Mux5/1 -> " 5"/2
  Manual Switch3/1 -> DM5/1(sig1)
  Manual Switch1/1 -> DM6/1(sig2)
  " 5"/1 -> Gain14/1
  Sum2/1 -> Mkudm/1

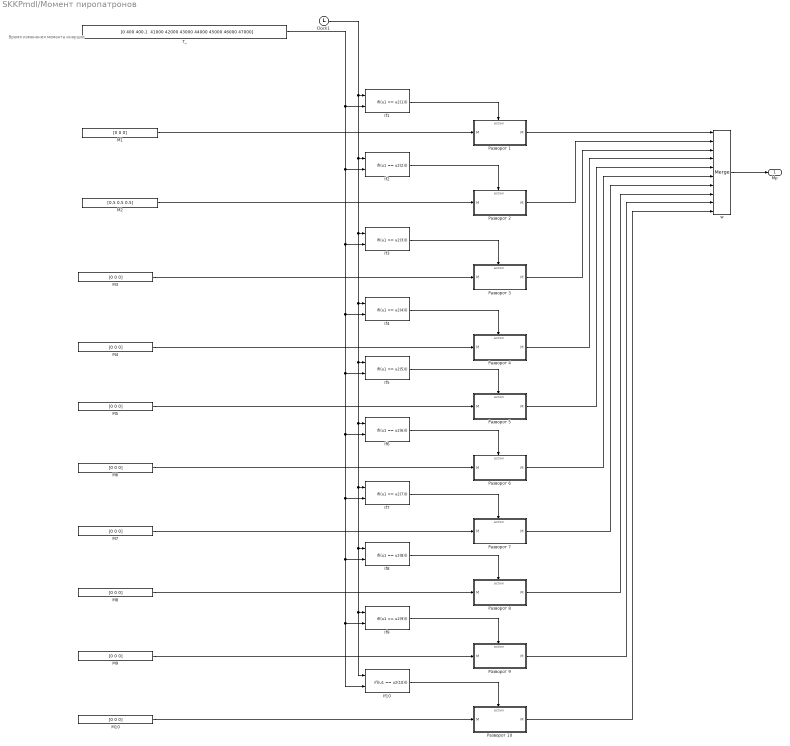
== system SKKPmdl/Момент пиропатронов ==
  note: Время изменения момента инерции
  Clock1 : Clock
  If1 : If  NumInputs=2  IfExpression=(u1 == u2(1))  ShowElse=off
  If10 : If  NumInputs=2  IfExpression=(u1 == u2(10))  ShowElse=off
  If2 : If  NumInputs=2  IfExpression=(u1 == u2(2))  ShowElse=off
  If3 : If  NumInputs=2  IfExpression=(u1 == u2(3))  ShowElse=off
  If4 : If  NumInputs=2  IfExpression=(u1 == u2(4))  ShowElse=off
  If5 : If  NumInputs=2  IfExpression=(u1 == u2(5))  ShowElse=off
  If6 : If  NumInputs=2  IfExpression=(u1 == u2(6))  ShowElse=off
  If7 : If  NumInputs=2  IfExpression=(u1 == u2(7))  ShowElse=off
  If8 : If  NumInputs=2  IfExpression=(u1 == u2(8))  ShowElse=off
  If9 : If  NumInputs=2  IfExpression=(u1 == u2(9))  ShowElse=off
  M{1,3..10} (9 alike) : Constant  Value=[0 0 0]
  M2 : Constant  Value=[0.5 0.5 0.5]
  T_ : Constant  Value="[0 400 400.1  41000 42000 43000 44000 45000 46000 47000]"
  "w " : Merge  Inputs=10
  Разворот 1 : Subsystem  TreatAsAtomicUnit=on
  Разворот 10 : Subsystem  TreatAsAtomicUnit=on
  Разворот 2 : Subsystem  TreatAsAtomicUnit=on
  Разворот 3 : Subsystem  TreatAsAtomicUnit=on
  Разворот 4 : Subsystem  TreatAsAtomicUnit=on
  Разворот 5 : Subsystem  TreatAsAtomicUnit=on
  Разворот 6 : Subsystem  TreatAsAtomicUnit=on
  Разворот 7 : Subsystem  TreatAsAtomicUnit=on
  Разворот 8 : Subsystem  TreatAsAtomicUnit=on
  Разворот 9 : Subsystem  TreatAsAtomicUnit=on
  Mp : Outport
  wires:
  M1/1 -> Разворот 1/1(M)
  If1/1 -> Разворот 1/Action
  M2/1 -> Разворот 2/1(M)
  If2/1 -> Разворот 2/Action
  M3/1 -> Разворот 3/1(M)
  If3/1 -> Разворот 3/Action
  M4/1 -> Разворот 4/1(M)
  If4/1 -> Разворот 4/Action
  M5/1 -> Разворот 5/1(M)
  If5/1 -> Разворот 5/Action
  M6/1 -> Разворот 6/1(M)
  If6/1 -> Разворот 6/Action
  M7/1 -> Разворот 7/1(M)
  If7/1 -> Разворот 7/Action
  M8/1 -> Разворот 8/1(M)
  If8/1 -> Разворот 8/Action
  M9/1 -> Разворот 9/1(M)
  If9/1 -> Разворот 9/Action
  M10/1 -> Разворот 10/1(M)
  If10/1 -> Разворот 10/Action
  Разворот 1/1("M ") -> "w "/1
  Разворот 2/1("M ") -> "w "/2
  Разворот 3/1("M ") -> "w "/3
  Разворот 4/1("M ") -> "w "/4
  Разворот 5/1("M ") -> "w "/5
  Разворот 6/1("M ") -> "w "/6
  Разворот 7/1("M ") -> "w "/7
  Разворот 8/1("M ") -> "w "/8
  Разворот 9/1("M ") -> "w "/9
  Разворот 10/1("M ") -> "w "/10
  T_/1 -> If2/2, If4/2, If6/2, If10/2, If9/2, If8/2, If7/2, If5/2, If3/2, If1/2
  Clock1/1 -> If10/1, If9/1, If8/1, If7/1, If6/1, If5/1, If4/1, If3/1, If2/1, If1/1
  "w "/1 -> Mp/1

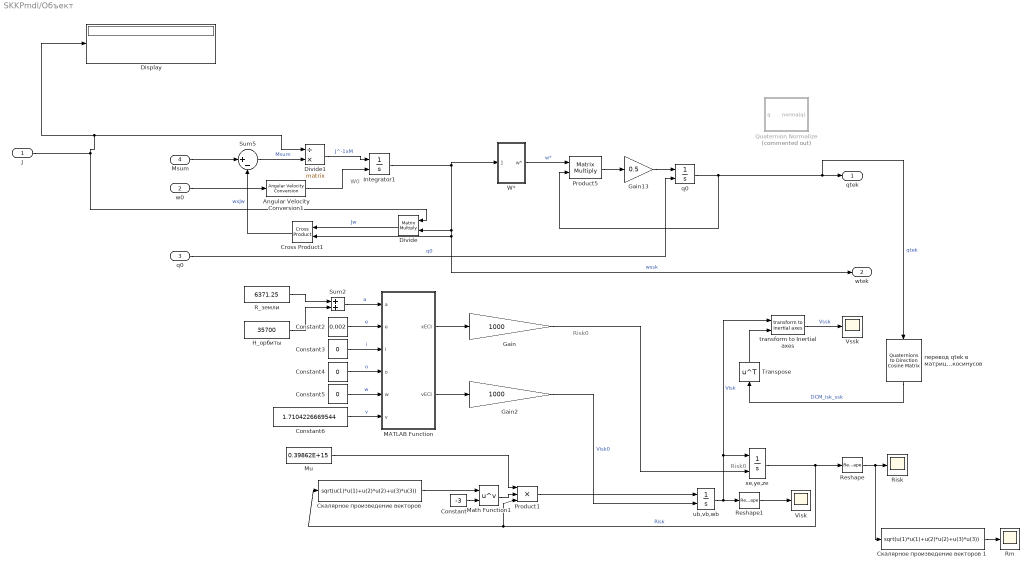
== system SKKPmdl/Объект ==
  note: Risk0
  note: W0
  note: Risk0
  J : Inport
  w0 : Inport  Port=2
  "q0 " : Inport  Port=3
  Msum : Inport  Port=4
  Angular Velocity Conversion1 : aerolibconvert2/Angular Velocity Conversion  IU=deg/s  OU=rad/s
  Constant : Constant  Value=-3
  Constant2 : Constant  Value=0.002
  Constant3 : Constant  Value=0
  Constant4 : Constant  Value=0
  Constant5 : Constant  Value=0
  Constant6 : Constant  Value=1.7104226669544
  Cross Product1 : vrlib/Utilities/Cross Product
  Display : Display
  Divide : Product  Inputs=**  Multiplication=Matrix(*)
  Divide1 : Product  Inputs=/*  Multiplication=Matrix(*)
  Gain : Gain  Gain=1000
  Gain13 : Gain  Gain=0.5
  Gain2 : Gain  Gain=1000
  H_орбиты : Constant  Value=35700
  Integrator1 : Integrator  InitialConditionSource=external
  MATLAB Function : MATLAB Function  TreatAsAtomicUnit=on
  Math Function1 : Math  Operator=pow  SaturateOnIntegerOverflow=on
  Mu : Constant  Value=0.39862E+15
  Product1 : Product  Inputs=3  SaturateOnIntegerOverflow=on  OutDataTypeStr=Inherit: Same as first input
  Product5 : Product  Multiplication=Matrix(*)  SaturateOnIntegerOverflow=on  OutDataTypeStr=Inherit: Same as first input
  "Quaternion Normalize " : Subsystem  Commented=on
  R_земли : Constant  Value=6371.25
  Reshape : Reshape
  Reshape1 : Reshape
  Risk : Scope
      settings: SaveName=Risk
  Rm : Scope
      settings: YMin=7e+06  YMax=7.8e+06  SaveName=Rm
  Sum2 : Sum  SaturateOnIntegerOverflow=on
  Sum5 : Sum  Inputs=|+-
  Transpose : Math  Operator=transpose  SaturateOnIntegerOverflow=on
  Visk : Scope
      settings: SaveName=Visk
  Vssk : Scope
      settings: SaveName=Vssk
  W* : Subsystem
  q0 : Integrator  InitialConditionSource=external
  "transform to Inertial axes " : aerolib6dof2/6DOF (Euler Angles)/transform to Inertial axes   SystemSampleTime=-1
  ub,vb,wb : Integrator  InitialConditionSource=external  InitialCondition=convvel(V0,'m/s','m/s')
  xe,ye,ze : Integrator  InitialConditionSource=external  InitialCondition=R0
  "Скалярное произведение векторов " : Fcn  Expr=sqrt(u(1)*u(1)+u(2)*u(2)+u(3)*u(3))
  Скалярное произведение векторов 1 : Fcn  Expr=sqrt(u(1)*u(1)+u(2)*u(2)+u(3)*u(3))
  "перевод qtek в матрицу направляющих косинусов " : aerolibtransform2/Quaternions to  Direction Cosine Matrix
  qtek : Outport
  wtek : Outport  Port=2
  wires:
  "transform to Inertial axes "/1 -> Vssk/1  "Vssk"
  xe,ye,ze/1 -> "Скалярное произведение векторов "/1, Product1/3, Reshape/1  "Risk"
  Sum2/1 -> MATLAB Function/1(a)  "a"
  H_орбиты/1 -> Sum2/2
  R_земли/1 -> Sum2/1
  Gain2/1 -> ub,vb,wb/2  "Visk0"
  Constant4/1 -> MATLAB Function/4(o)  "o"
  Constant2/1 -> MATLAB Function/2(e)  "e"
  Constant3/1 -> MATLAB Function/3(i)  "i"
  Constant5/1 -> MATLAB Function/5(w)  "w"
  Constant6/1 -> MATLAB Function/6(v)  "v"
  MATLAB Function/1(xECI) -> Gain/1
  MATLAB Function/2(vECI) -> Gain2/1
  Mu/1 -> Product1/1
  Math Function1/1 -> Product1/2
  Constant/1 -> Math Function1/2
  "перевод qtek в матрицу направляющих косинусов "/1 -> Transpose/1  "DCM_isk_ssk"
  Transpose/1 -> "transform to Inertial axes "/2
  ub,vb,wb/1 -> Reshape1/1, xe,ye,ze/1, "transform to Inertial axes "/1  "Visk"
  Product1/1 -> ub,vb,wb/1
  W*/1(w*) -> Product5/1  "w*"
  "q0 "/1 -> q0/2  "q0"
  Msum/1 -> Sum5/1
  Divide/1 -> Cross Product1/1  "Jw"
  Sum5/1 -> Divide1/2  "Msum"
  Cross Product1/1 -> Sum5/2  "wxJw"
  Angular Velocity Conversion1/1 -> Integrator1/2
  Divide1/1 -> Integrator1/1  "J^-1xM"
  Product5/1 -> Gain13/1
  Gain13/1 -> q0/1
  w0/1 -> Angular Velocity Conversion1/1
  "Скалярное произведение векторов "/1 -> Math Function1/1
  Gain/1 -> xe,ye,ze/2
  Reshape/1 -> Скалярное произведение векторов 1/1, Risk/1
  Reshape1/1 -> Visk/1
  Скалярное произведение векторов 1/1 -> Rm/1
  q0/1 -> qtek/1, "перевод qtek в матрицу направляющих косинусов "/1, Product5/2  "qtek"
  J/1 -> Divide1/1, Display/1, Divide/1
  Integrator1/1 -> W*/1(wssk), Divide/2, Cross Product1/2, wtek/1  "wssk"

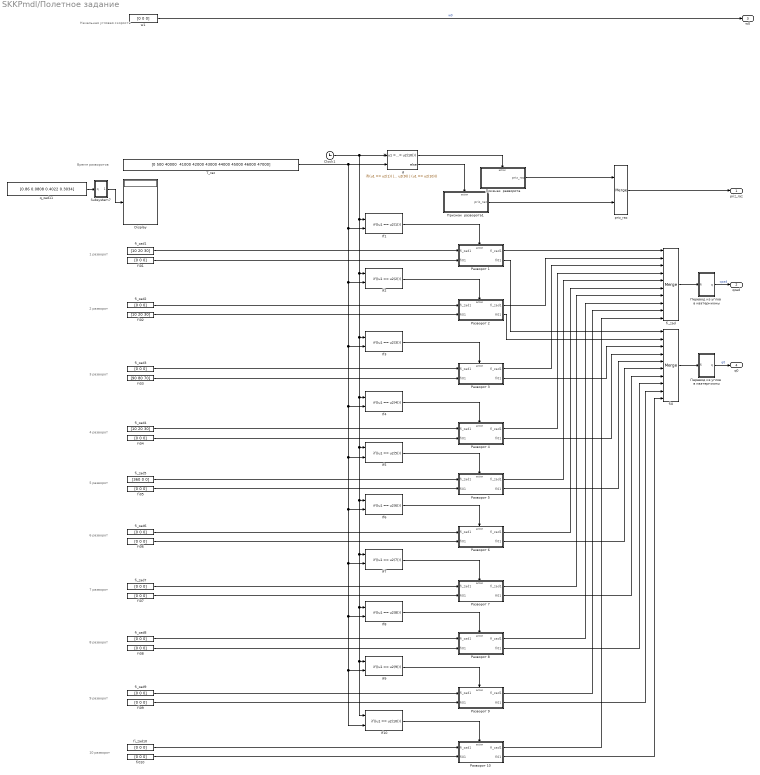
== system SKKPmdl/Полетное задание ==
  note: Начальная угловая скорость
  note: Время разворотов
  note: 10 разворот
  note: 9 разворот
  note: 8 разворот
  note: 7 разворот
  note: 6 разворот
  note: 5 разворот
  note: 4 разворот
  note: 3 разворот
  note: 2 разворот
  note: 1 разворот
  Clock1 : Clock
  Display : Display
  If : If  NumInputs=2  IfExpression=(u1 == u2(1)) | (u1 == u2(2)) | (u1 == u2(3)) | (u1 == u2(4)) | (u1 == u2(5)) | (u1 == u2(6)) | (u1 == u2(7)) | (u1 == u2(8)) | (u1 == u2(9)) | (u1 == u2(10))
  If1 : If  NumInputs=2  IfExpression=(u1 == u2(1))  ShowElse=off
  If10 : If  NumInputs=2  IfExpression=(u1 == u2(10))  ShowElse=off
  If2 : If  NumInputs=2  IfExpression=(u1 == u2(2))  ShowElse=off
  If3 : If  NumInputs=2  IfExpression=(u1 == u2(3))  ShowElse=off
  If4 : If  NumInputs=2  IfExpression=(u1 == u2(4))  ShowElse=off
  If5 : If  NumInputs=2  IfExpression=(u1 == u2(5))  ShowElse=off
  If6 : If  NumInputs=2  IfExpression=(u1 == u2(6))  ShowElse=off
  If7 : If  NumInputs=2  IfExpression=(u1 == u2(7))  ShowElse=off
  If8 : If  NumInputs=2  IfExpression=(u1 == u2(8))  ShowElse=off
  If9 : If  NumInputs=2  IfExpression=(u1 == u2(9))  ShowElse=off
  Subsystem7 : Subsystem
  T_raz : Constant  Value="[0 500 40000  41000 42000 43000 44000 45000 46000 47000]"
  fi0 : Merge  Inputs=10
  fi01 : Constant  Value=[0 0 0]
  fi010 : Constant  Value=[0 0 0]
  fi02 : Constant  Value=[10 20 30]
  fi03 : Constant  Value=[90 80 70]
  fi04 : Constant  Value=[0 0 0]
  fi05 : Constant  Value=[0 0 0]
  fi06 : Constant  Value=[0 0 0]
  fi07 : Constant  Value=[0 0 0]
  fi08 : Constant  Value=[0 0 0]
  fi09 : Constant  Value=[0 0 0]
  fi_zad : Merge  Inputs=10
  fi_zad1 : Constant  Value=[10 20 30]
  fi_zad{2..3,6..10} (7 alike) : Constant  Value=[0 0 0]
  fi_zad4 : Constant  Value=[10 20 30]
  fi_zad5 : Constant  Value=[360 0 0]
  "priz_raz " : Merge
  q_zad11 : Constant  Value=[0.86 0.0808 0.4022 0.3034]
  w1 : Constant  Value=[0 0 0]
  Перевод из углов  в кватернионы : Subsystem
  "Перевод из углов  в кватернионы " : Subsystem
  Признак  разворота : Subsystem  TreatAsAtomicUnit=on
  Признак  разворота1 : Subsystem  TreatAsAtomicUnit=on
  Разворот 1 : Subsystem  TreatAsAtomicUnit=on
  Разворот 10 : Subsystem  TreatAsAtomicUnit=on
  Разворот 2 : Subsystem  TreatAsAtomicUnit=on
  Разворот 3 : Subsystem  TreatAsAtomicUnit=on
  Разворот 4 : Subsystem  TreatAsAtomicUnit=on
  Разворот 5 : Subsystem  TreatAsAtomicUnit=on
  Разворот 6 : Subsystem  TreatAsAtomicUnit=on
  Разворот 7 : Subsystem  TreatAsAtomicUnit=on
  Разворот 8 : Subsystem  TreatAsAtomicUnit=on
  Разворот 9 : Subsystem  TreatAsAtomicUnit=on
  priz_raz : Outport
  qzad : Outport  Port=2
  w0 : Outport  Port=3
  q0 : Outport  Port=4
  wires:
  Subsystem7/1(deg) -> Display/1
  q_zad11/1 -> Subsystem7/1(q)
  "priz_raz "/1 -> priz_raz/1
  If/2 -> Признак  разворота1/Action
  Признак  разворота1/1(priz_raz) -> "priz_raz "/2
  fi0/1 -> "Перевод из углов  в кватернионы "/1(fi)
  fi_zad/1 -> Перевод из углов  в кватернионы/1(fi)
  Clock1/1 -> If/1, If1/1, If2/1, If3/1, If4/1, If5/1, If6/1, If7/1, If8/1, If9/1, If10/1
  T_raz/1 -> If/2, If1/2, If3/2, If5/2, If7/2, If8/2, If9/2, If10/2, If6/2, If4/2, If2/2
  "Перевод из углов  в кватернионы "/1(q) -> q0/1  "q0"
  Перевод из углов  в кватернионы/1(q) -> qzad/1  "qzad"
  Разворот 10/2("fi01  ") -> fi0/10
  Разворот 9/2("fi01  ") -> fi0/9
  Разворот 8/2("fi01  ") -> fi0/8
  Разворот 7/2("fi01  ") -> fi0/7
  Разворот 6/2("fi01  ") -> fi0/6
  Разворот 5/2("fi01  ") -> fi0/5
  Разворот 4/2("fi01  ") -> fi0/4
  Разворот 3/2("fi01  ") -> fi0/3
  Разворот 2/2("fi01  ") -> fi0/2
  Разворот 10/1("fi_zad1  ") -> fi_zad/10
  Разворот 9/1("fi_zad1  ") -> fi_zad/9
  Разворот 8/1("fi_zad1  ") -> fi_zad/8
  Разворот 7/1("fi_zad1  ") -> fi_zad/7
  Разворот 6/1("fi_zad1  ") -> fi_zad/6
  Разворот 5/1("fi_zad1  ") -> fi_zad/5
  Разворот 4/1("fi_zad1  ") -> fi_zad/4
  Разворот 3/1("fi_zad1  ") -> fi_zad/3
  Разворот 2/1("fi_zad1  ") -> fi_zad/2
  Разворот 1/2("fi01  ") -> fi0/1
  Разворот 1/1("fi_zad1  ") -> fi_zad/1
  If10/1 -> Разворот 10/Action
  fi_zad10/1 -> Разворот 10/1(fi_zad1)
  fi010/1 -> Разворот 10/2(fi01)
  If9/1 -> Разворот 9/Action
  fi_zad9/1 -> Разворот 9/1(fi_zad1)
  fi09/1 -> Разворот 9/2(fi01)
  If8/1 -> Разворот 8/Action
  fi_zad8/1 -> Разворот 8/1(fi_zad1)
  fi08/1 -> Разворот 8/2(fi01)
  If7/1 -> Разворот 7/Action
  fi_zad7/1 -> Разворот 7/1(fi_zad1)
  fi07/1 -> Разворот 7/2(fi01)
  If6/1 -> Разворот 6/Action
  fi_zad6/1 -> Разворот 6/1(fi_zad1)
  fi06/1 -> Разворот 6/2(fi01)
  If5/1 -> Разворот 5/Action
  fi_zad5/1 -> Разворот 5/1(fi_zad1)
  fi05/1 -> Разворот 5/2(fi01)
  If4/1 -> Разворот 4/Action
  fi_zad4/1 -> Разворот 4/1(fi_zad1)
  fi04/1 -> Разворот 4/2(fi01)
  If3/1 -> Разворот 3/Action
  fi_zad3/1 -> Разворот 3/1(fi_zad1)
  fi03/1 -> Разворот 3/2(fi01)
  If2/1 -> Разворот 2/Action
  fi_zad2/1 -> Разворот 2/1(fi_zad1)
  fi02/1 -> Разворот 2/2(fi01)
  If1/1 -> Разворот 1/Action
  fi_zad1/1 -> Разворот 1/1(fi_zad1)
  fi01/1 -> Разворот 1/2(fi01)
  Признак  разворота/1(priz_raz) -> "priz_raz "/1
  If/1 -> Признак  разворота/Action
  w1/1 -> w0/1  "w0"

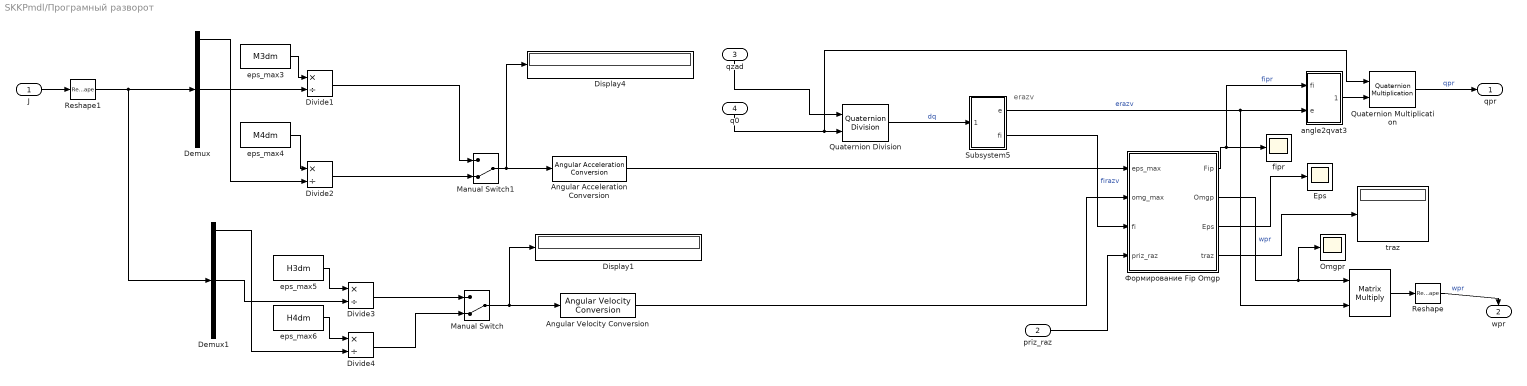
== system SKKPmdl/Програмный разворот  ==
  note: erazv
  J : Inport
  priz_raz : Inport  Port=2
  qzad : Inport  Port=3
  q0 : Inport  Port=4
  "  " : Product  Multiplication=Matrix(*)  SaturateOnIntegerOverflow=on  RndMeth=Zero  InputSameDT=on  OutDataTypeStr=Inherit: Same as first input
  Angular Acceleration Conversion : aerolibconvert2/Angular Acceleration Conversion  IU=rad/s^2  OU=deg/s^2
  Angular Velocity Conversion : aerolibconvert2/Angular Velocity Conversion  IU=rad/s  OU=deg/s
  Demux : Demux  Outputs=9
  Demux1 : Demux  Outputs=9
  Display1 : Display
  Display4 : Display
  Divide{1..4} (4 alike) : Product  Inputs=*/
  Eps : Scope
      settings: YMin=-0.01  YMax=0.01
  Manual Switch : ManualSwitch  CurrentSetting=0
  Manual Switch1 : ManualSwitch  CurrentSetting=0
  Omgpr : Scope
      settings: YMin=-0.1  YMax=0.3  SaveName=ScopeData10
  Quaternion Division : aerolibutil/Quaternion Division
  Quaternion Multiplication : aerolibutil/Quaternion Multiplication
  Reshape : Reshape
  Reshape1 : Reshape  OutputDimensionality=Column vector (2-D)
  Subsystem5 : Subsystem
  angle2qvat3 : Subsystem
  eps_max3 : Constant  Value=M3dm
  eps_max4 : Constant  Value=M4dm
  eps_max5 : Constant  Value=H3dm
  eps_max6 : Constant  Value=H4dm
  fipr : Scope
      settings: YMin=0  YMax=40  SaveName=ScopeData20
  traz : Display
  Формирование Fip Omgp : Stateflow chart  TreatAsAtomicUnit=on
  qpr : Outport
  wpr : Outport  Port=2
  wires:
  Subsystem5/2(fi) -> Формирование Fip Omgp/3(fi)  "firazv"
  Subsystem5/1(e) -> "  "/2, angle2qvat3/2(e)  "erazv"
  Quaternion Division/1 -> Subsystem5/1(qvat)  "dq"
  Формирование Fip Omgp/2(Omgp) -> Omgpr/1, "  "/1  "wpr"
  angle2qvat3/1(Quat) -> Quaternion Multiplication/2
  "  "/1 -> Reshape/1
  Reshape/1 -> wpr/1  "wpr"
  Quaternion Multiplication/1 -> qpr/1  "qpr"
  priz_raz/1 -> Формирование Fip Omgp/4(priz_raz)
  qzad/1 -> Quaternion Division/1
  q0/1 -> Quaternion Division/2, Quaternion Multiplication/1
  Формирование Fip Omgp/4(traz) -> traz/1
  Формирование Fip Omgp/3(Eps) -> Eps/1
  Manual Switch1/1 -> Display4/1, Angular Acceleration Conversion/1
  Divide3/1 -> Manual Switch/1
  Manual Switch/1 -> Display1/1, Angular Velocity Conversion/1
  Divide4/1 -> Manual Switch/2
  Divide2/1 -> Manual Switch1/2
  Формирование Fip Omgp/1(Fip) -> angle2qvat3/1(fi), fipr/1  "fipr"
  Divide1/1 -> Manual Switch1/1
  Angular Acceleration Conversion/1 -> Формирование Fip Omgp/1(eps_max)
  Angular Velocity Conversion/1 -> Формирование Fip Omgp/2(omg_max)
  Demux/5 -> Divide1/2
  Demux/1 -> Divide2/2
  eps_max3/1 -> Divide1/1
  eps_max4/1 -> Divide2/1
  Demux1/5 -> Divide3/2
  Demux1/1 -> Divide4/2
  eps_max5/1 -> Divide3/1
  eps_max6/1 -> Divide4/1
  J/1 -> Reshape1/1
  Reshape1/1 -> Demux/1, Demux1/1

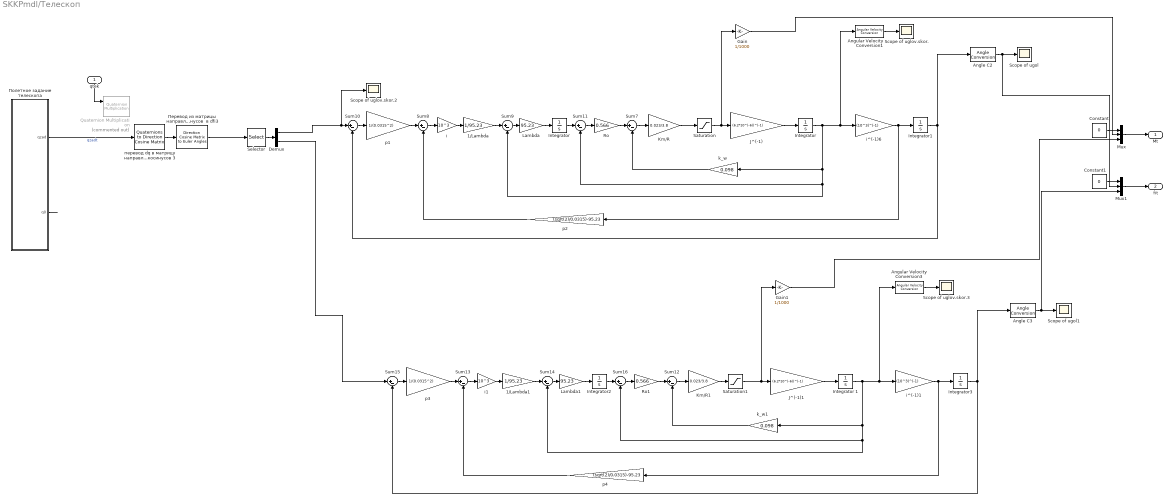
== system SKKPmdl/Телескоп ==
  qtek : Inport
  1/Lambda : Gain  Gain=1/95.23  SaturateOnIntegerOverflow=on  OutDataTypeStr=Inherit: Same as input  ParamDataTypeStr=Inherit: Same as input
  1/Lambda1 : Gain  Gain=1/95.23  SaturateOnIntegerOverflow=on  OutDataTypeStr=Inherit: Same as input  ParamDataTypeStr=Inherit: Same as input
  Angle C2 : aerolibconvert2/Angle Conversion  IU=rad  OU=deg
  Angle C3 : aerolibconvert2/Angle Conversion  IU=rad  OU=deg
  Angular Velocity Conversion1 : aerolibconvert2/Angular Velocity Conversion  IU=rad/s  OU=deg/s
  Angular Velocity Conversion3 : aerolibconvert2/Angular Velocity Conversion  IU=rad/s  OU=deg/s
  Constant : Constant  Value=0
  Constant1 : Constant  Value=0
  Demux : Demux  Outputs=2
  Gain : Gain  Gain=1/1000
  Gain1 : Gain  Gain=1/1000
  Integrator{,1..3} (4 alike) : Integrator
  "Integrator " : Integrator
  Integrator 1 : Integrator
  J^(-1) : Gain  Gain=(6.2*10^(-6))^(-1)  SaturateOnIntegerOverflow=on  OutDataTypeStr=Inherit: Same as input  ParamDataTypeStr=Inherit: Same as input
  J^(-1)1 : Gain  Gain=(6.2*10^(-6))^(-1)  SaturateOnIntegerOverflow=on  OutDataTypeStr=Inherit: Same as input  ParamDataTypeStr=Inherit: Same as input
  Km/R : Gain  Gain=0.023/3.8  SaturateOnIntegerOverflow=on  OutDataTypeStr=Inherit: Same as input  ParamDataTypeStr=Inherit: Same as input
  Km/R1 : Gain  Gain=0.023/3.8  SaturateOnIntegerOverflow=on  OutDataTypeStr=Inherit: Same as input  ParamDataTypeStr=Inherit: Same as input
  Lambda : Gain  Gain=95.23  SaturateOnIntegerOverflow=on  OutDataTypeStr=Inherit: Same as input  ParamDataTypeStr=Inherit: Same as input
  Lambda1 : Gain  Gain=95.23  SaturateOnIntegerOverflow=on  OutDataTypeStr=Inherit: Same as input  ParamDataTypeStr=Inherit: Same as input
  Mux : Mux  Inputs=3
  Mux1 : Mux  Inputs=3
  Quaternion Multiplication : aerolibutil/Quaternion Multiplication  Commented=on
  Ro : Gain  Gain=0.566  SaturateOnIntegerOverflow=on  OutDataTypeStr=Inherit: Same as input  ParamDataTypeStr=Inherit: Same as input
  Ro1 : Gain  Gain=0.566  SaturateOnIntegerOverflow=on  OutDataTypeStr=Inherit: Same as input  ParamDataTypeStr=Inherit: Same as input
  Saturation : Saturate  UpperLimit=7.85  LowerLimit=-7.85
  Saturation1 : Saturate  UpperLimit=7.85  LowerLimit=-7.85
  Scope of uglov.skor. : Scope
      settings: TickLabels=on  TimeRange=3  YMin=-500  YMax=2000  SaveName=ScopeData3  MaxDataPoints=50000
  Scope of uglov.skor.2 : Scope
      settings: TickLabels=on  TimeRange=3  YMin=0.15  YMax=0.55  SaveName=ScopeData6  MaxDataPoints=50000
  Scope of uglov.skor.3 : Scope
      settings: TickLabels=on  TimeRange=3  YMin=-500  YMax=2000  MaxDataPoints=50000
  Scope of ugol : Scope
      settings: TickLabels=on  TimeRange=14.02635825712749  YMin=-4000  YMax=4000  SaveName=ScopeData4  MaxDataPoints=50000
  Scope of ugol1 : Scope
      settings: TickLabels=on  TimeRange=14.02635825712749  YMin=5  YMax=35  SaveName=ScopeData9  MaxDataPoints=50000
  Selector : Selector  InputPortWidth=3  Indices=[2 3]
  Sum{7..16} (10 alike) : Sum  Inputs=|+-
  i : Gain  Gain=10^3  SaturateOnIntegerOverflow=on  OutDataTypeStr=Inherit: Same as input  ParamDataTypeStr=Inherit: Same as input
  i1 : Gain  Gain=10^3  SaturateOnIntegerOverflow=on  OutDataTypeStr=Inherit: Same as input  ParamDataTypeStr=Inherit: Same as input
  i^(-1)1 : Gain  Gain=(10^3)^(-1)  SaturateOnIntegerOverflow=on  OutDataTypeStr=Inherit: Same as input  ParamDataTypeStr=Inherit: Same as input
  i^(-1)6 : Gain  Gain=(10^3)^(-1)  SaturateOnIntegerOverflow=on  OutDataTypeStr=Inherit: Same as input  ParamDataTypeStr=Inherit: Same as input
  k_w : Gain  Gain=0.098  SaturateOnIntegerOverflow=on  OutDataTypeStr=Inherit: Same as input  ParamDataTypeStr=Inherit: Same as input
  k_w1 : Gain  Gain=0.098  SaturateOnIntegerOverflow=on  OutDataTypeStr=Inherit: Same as input  ParamDataTypeStr=Inherit: Same as input
  p1 : Gain  Gain=1/(0.0315^2)  SaturateOnIntegerOverflow=on  OutDataTypeStr=Inherit: Same as input  ParamDataTypeStr=Inherit: Same as input
  p2 : Gain  Gain=(sqrt(2)/0.0315)-95.23  SaturateOnIntegerOverflow=on  OutDataTypeStr=Inherit: Same as input  ParamDataTypeStr=Inherit: Same as input
  p3 : Gain  Gain=1/(0.0315^2)  SaturateOnIntegerOverflow=on  OutDataTypeStr=Inherit: Same as input  ParamDataTypeStr=Inherit: Same as input
  p4 : Gain  Gain=(sqrt(2)/0.0315)-95.23  SaturateOnIntegerOverflow=on  OutDataTypeStr=Inherit: Same as input  ParamDataTypeStr=Inherit: Same as input
  Перевод из матрицы направляющих косинусов  в dfi3 : aerolibobsolete/Direction Cosine Matrix to Euler Angles
  Полетное задание телескопа : Subsystem
  перевод dq в матрицу направляющих косинусов 3 : aerolibtransform2/Quaternions to  Direction Cosine Matrix
  Mt : Outport
  fit : Outport  Port=2
  wires:
  Selector/1 -> Demux/1
  Sum10/1 -> p1/1
  p1/1 -> Sum8/1
  k_w/1 -> Sum7/2
  "Integrator "/1 -> i^(-1)6/1, Angular Velocity Conversion1/1, Sum11/2, Sum9/2, k_w/1
  Integrator1/1 -> Sum10/2, Angle C2/1
  Sum8/1 -> i/1
  Sum9/1 -> Lambda/1
  Lambda/1 -> Integrator/1
  p2/1 -> Sum8/2
  i^(-1)6/1 -> p2/1, Integrator1/1
  Demux/1 -> Scope of uglov.skor.2/1, Sum10/1
  Angle C2/1 -> Mux1/2, Scope of ugol/1
  1/Lambda/1 -> Sum9/1
  Angular Velocity Conversion1/1 -> Scope of uglov.skor./1
  Ro/1 -> Sum7/1
  i/1 -> 1/Lambda/1
  Sum11/1 -> Ro/1
  Sum7/1 -> Km/R/1
  J^(-1)/1 -> "Integrator "/1
  Km/R/1 -> Saturation/1
  Integrator/1 -> Sum11/1
  Saturation1/1 -> Gain1/1, J^(-1)1/1
  Sum15/1 -> p3/1
  Перевод из матрицы направляющих косинусов  в dfi3/1 -> Selector/1
  p3/1 -> Sum13/1
  Integrator3/1 -> Sum15/2, Angle C3/1
  i1/1 -> 1/Lambda1/1
  Sum14/1 -> Lambda1/1
  Sum16/1 -> Ro1/1
  Lambda1/1 -> Integrator2/1
  p4/1 -> Sum13/2
  Integrator2/1 -> Sum16/1
  Sum12/1 -> Km/R1/1
  k_w1/1 -> Sum12/2
  Ro1/1 -> Sum12/1
  Integrator 1/1 -> i^(-1)1/1, Angular Velocity Conversion3/1, Sum16/2, Sum14/2, k_w1/1
  J^(-1)1/1 -> Integrator 1/1
  i^(-1)1/1 -> p4/1, Integrator3/1
  1/Lambda1/1 -> Sum14/1
  Angle C3/1 -> Mux1/3, Scope of ugol1/1
  Angular Velocity Conversion3/1 -> Scope of uglov.skor.3/1
  Km/R1/1 -> Saturation1/1
  Sum13/1 -> i1/1
  перевод dq в матрицу направляющих косинусов 3/1 -> Перевод из матрицы направляющих косинусов  в dfi3/1
  Gain1/1 -> Mux/3
  Gain/1 -> Mux/2
  Полетное задание телескопа/1(qzad) -> перевод dq в матрицу направляющих косинусов 3/1  "qzadt"
  Saturation/1 -> Gain/1, J^(-1)/1
  Полетное задание телескопа/2(q0) -> ?
  qtek/1 -> Quaternion Multiplication/1
  Constant/1 -> Mux/1
  Constant1/1 -> Mux1/1
  Mux1/1 -> fit/1
  Mux/1 -> Mt/1
  Demux/2 -> Sum15/1
